simulink subsystem "PID"  (R2023b)
settings: Solver=VariableStepAuto  StartTime=0.0  StopTime=10.0  RelTol=1e-3
undefined symbols (not defined in the file): kd, ki, kp
settings Model: Creator=tomasz  LastModifiedBy=tomasz

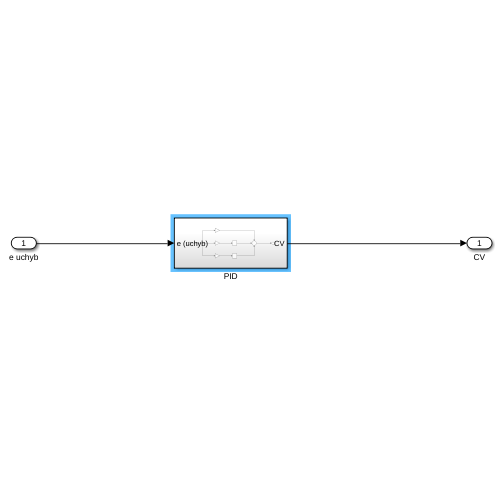
[thumbnail: Simulink's stored preview of the top-level diagram]
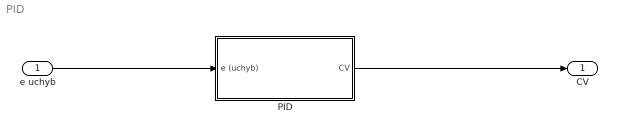
== system PID ==
  e uchyb : Inport
  PID : Subsystem
  CV : Outport
  wires:
  e uchyb/1 -> PID/1(e (uchyb))
  PID/1(CV) -> CV/1

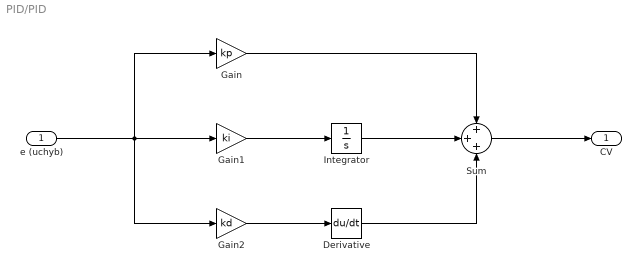
== system PID/PID ==
  e (uchyb) : Inport
  Derivative : Derivative
  Gain : Gain  Gain=kp
  Gain1 : Gain  Gain=ki
  Gain2 : Gain  Gain=kd
  Integrator : Integrator
  Sum : Sum  Inputs=+++
  CV : Outport
  wires:
  Integrator/1 -> Sum/2
  Gain2/1 -> Derivative/1
  Gain1/1 -> Integrator/1
  Gain/1 -> Sum/1
  e (uchyb)/1 -> Gain1/1, Gain/1, Gain2/1
  Derivative/1 -> Sum/3
  Sum/1 -> CV/1
